simulink model "K_Sim"  (R2020b)
settings: Solver=FixedStepAuto  StartTime=0  StopTime=5  FixedStep=Ts  RelTol=1e-3
undefined symbols (not defined in the file or in its folder): DeviceDiscreDamping, DevicePara, DevicePowerFlow, DeviceType, Fbase, OtherInputs, Sbase, Ts, Vbase, Wbase, x_e, Ybase, Zbase
libraries: powerlib x264, SimplexPS x128
(part 2 of 2)

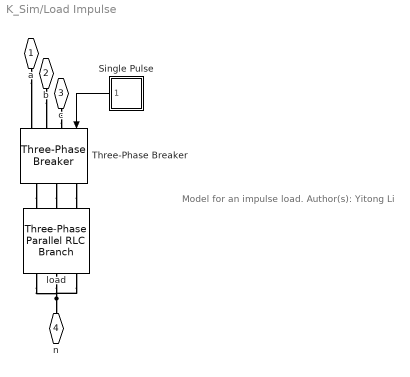
== system K_Sim/Load Impulse ==
  note: Model for an impulse load.
      |
      | Author(s): Yitong Li
  Single Pulse : Subsystem  AncestorBlock=SimplexPS/Single Pulse  mask{t0=t0, dt=dt, Am=1}
      mask prompts: t0 "t0 (s), starting time"; dt "dt (s), pulse width"; Am "Am, pulse amplitude"
  Three-Phase Breaker : powerlib/Elements/Three-Phase Breaker  InitialState=open  SwitchA=on  SwitchB=on  SwitchC=on  SwitchTimes="[1/60  5/60]"  External=on  BreakerResistance=0.01  SnubberResistance=1e6  SnubberCapacitance=inf  Measurements=None
  load : powerlib/Elements/Three-Phase Parallel RLC Branch  LConnTagsString=A|B|C  RConnTagsString=A|B|C  BranchType=R  Resistance=R  Inductance=1  Capacitance=1  Measurements=None
      settings: SourceProductBaseCode=PS
  a : PMIOPort  Side=Left
  b : PMIOPort  Port=2  Side=Left
  c : PMIOPort  Port=3  Side=Left
  n : PMIOPort  Port=4  Side=Right
  wires:
  Single Pulse/1(Out) -> Three-Phase Breaker/1
  connections:
  a/RConn1 -- Three-Phase Breaker/LConn3
  b/RConn1 -- Three-Phase Breaker/LConn2
  c/RConn1 -- Three-Phase Breaker/LConn1
  Three-Phase Breaker/RConn3 -- load/LConn1
  Three-Phase Breaker/RConn2 -- load/LConn2
  Three-Phase Breaker/RConn1 -- load/LConn3
  n/RConn1 -- load/RConn1 -- load/RConn3 -- load/RConn2

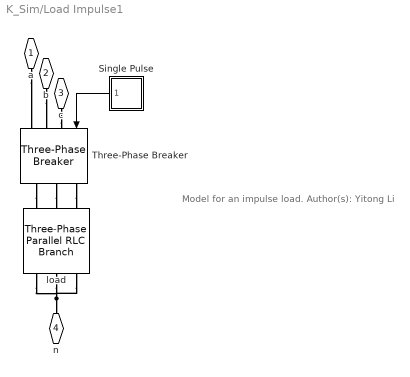
== system K_Sim/Load Impulse1 ==
  note: Model for an impulse load.
      |
      | Author(s): Yitong Li
  Single Pulse : Subsystem  AncestorBlock=SimplexPS/Single Pulse  mask{t0=t0, dt=dt, Am=1}
      mask prompts: t0 "t0 (s), starting time"; dt "dt (s), pulse width"; Am "Am, pulse amplitude"
  Three-Phase Breaker : powerlib/Elements/Three-Phase Breaker  InitialState=open  SwitchA=on  SwitchB=on  SwitchC=on  SwitchTimes="[1/60  5/60]"  External=on  BreakerResistance=0.01  SnubberResistance=1e6  SnubberCapacitance=inf  Measurements=None
  load : powerlib/Elements/Three-Phase Parallel RLC Branch  LConnTagsString=A|B|C  RConnTagsString=A|B|C  BranchType=R  Resistance=R  Inductance=1  Capacitance=1  Measurements=None
      settings: SourceProductBaseCode=PS
  a : PMIOPort  Side=Left
  b : PMIOPort  Port=2  Side=Left
  c : PMIOPort  Port=3  Side=Left
  n : PMIOPort  Port=4  Side=Right
  wires:
  Single Pulse/1(Out) -> Three-Phase Breaker/1
  connections:
  a/RConn1 -- Three-Phase Breaker/LConn3
  b/RConn1 -- Three-Phase Breaker/LConn2
  c/RConn1 -- Three-Phase Breaker/LConn1
  Three-Phase Breaker/RConn3 -- load/LConn1
  Three-Phase Breaker/RConn2 -- load/LConn2
  Three-Phase Breaker/RConn1 -- load/LConn3
  n/RConn1 -- load/RConn1 -- load/RConn3 -- load/RConn2

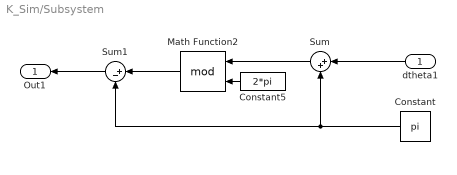
== system K_Sim/Subsystem ==
  dtheta1 : Inport
  Constant : Constant  Value=pi
  Constant5 : Constant  Value=2*pi
  Math Function2 : Math  Operator=mod  SignedPower=on  SaturateOnIntegerOverflow=on
  Sum : Sum  Inputs=|++
  Sum1 : Sum  Inputs=|+-
  Out1 : Outport
  wires:
  Constant5/1 -> Math Function2/2
  dtheta1/1 -> Sum/1
  Sum/1 -> Math Function2/1
  Math Function2/1 -> Sum1/1
  Sum1/1 -> Out1/1
  Constant/1 -> Sum1/2, Sum/2

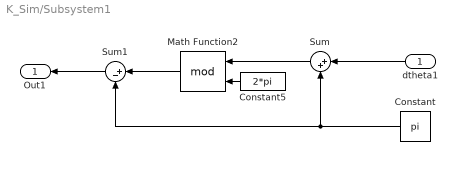
== system K_Sim/Subsystem1 ==
  dtheta1 : Inport
  Constant : Constant  Value=pi
  Constant5 : Constant  Value=2*pi
  Math Function2 : Math  Operator=mod  SignedPower=on  SaturateOnIntegerOverflow=on
  Sum : Sum  Inputs=|++
  Sum1 : Sum  Inputs=|+-
  Out1 : Outport
  wires:
  Constant5/1 -> Math Function2/2
  dtheta1/1 -> Sum/1
  Sum/1 -> Math Function2/1
  Math Function2/1 -> Sum1/1
  Sum1/1 -> Out1/1
  Constant/1 -> Sum1/2, Sum/2

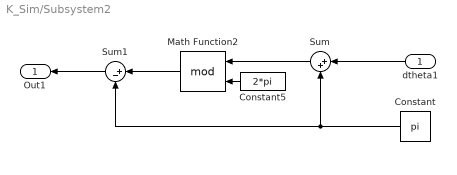
== system K_Sim/Subsystem2 ==
  dtheta1 : Inport
  Constant : Constant  Value=pi
  Constant5 : Constant  Value=2*pi
  Math Function2 : Math  Operator=mod  SignedPower=on  SaturateOnIntegerOverflow=on
  Sum : Sum  Inputs=|++
  Sum1 : Sum  Inputs=|+-
  Out1 : Outport
  wires:
  Constant5/1 -> Math Function2/2
  dtheta1/1 -> Sum/1
  Sum/1 -> Math Function2/1
  Math Function2/1 -> Sum1/1
  Sum1/1 -> Out1/1
  Constant/1 -> Sum1/2, Sum/2

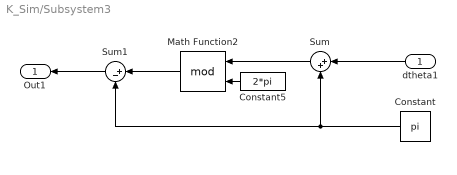
== system K_Sim/Subsystem3 ==
  dtheta1 : Inport
  Constant : Constant  Value=pi
  Constant5 : Constant  Value=2*pi
  Math Function2 : Math  Operator=mod  SignedPower=on  SaturateOnIntegerOverflow=on
  Sum : Sum  Inputs=|++
  Sum1 : Sum  Inputs=|+-
  Out1 : Outport
  wires:
  Constant5/1 -> Math Function2/2
  dtheta1/1 -> Sum/1
  Sum/1 -> Math Function2/1
  Math Function2/1 -> Sum1/1
  Sum1/1 -> Out1/1
  Constant/1 -> Sum1/2, Sum/2

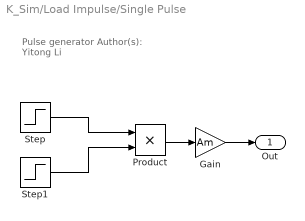
== system K_Sim/Load Impulse/Single Pulse ==
  note: Pulse generator
      |
      | Author(s): Yitong Li
  Gain : Gain  Gain=Am
  Product : Product
  Step : Step  Time=t0  SampleTime=0
  Step1 : Step  Time=t0+dt  Before=1  After=0  SampleTime=0
  Out : Outport
  wires:
  Gain/1 -> Out/1
  Product/1 -> Gain/1
  Step/1 -> Product/1
  Step1/1 -> Product/2

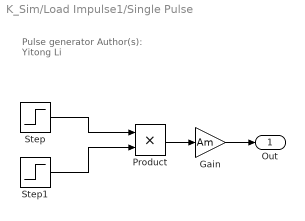
== system K_Sim/Load Impulse1/Single Pulse ==
  note: Pulse generator
      |
      | Author(s): Yitong Li
  Gain : Gain  Gain=Am
  Product : Product
  Step : Step  Time=t0  SampleTime=0
  Step1 : Step  Time=t0+dt  Before=1  After=0  SampleTime=0
  Out : Outport
  wires:
  Gain/1 -> Out/1
  Product/1 -> Gain/1
  Step/1 -> Product/1
  Step1/1 -> Product/2
